simulink model "compilation_1_sm_computation"  (Simulink 7.8)
settings: Solver=ode4  StartTime=0.0  StopTime=inf  FixedStep=0.001  RelTol=1e-3
libraries: opal_lib x6
Description:
  | Model of a simple control system for use iin training.
settings Model: Creator=Paul Baracos  LastModifiedBy=emma
settings DataIOCC: SaveOutput=off  SaveTime=off  SignalLoggingName=sigsOut
settings OptimizationCC: BlockReduction=off  BooleanDataType=off  InlineInvariantSignals=on  InitFltsAndDblsToZero=on
settings DebuggingCC: SaveWithParameterizedLinksMsg=none  SignalResolutionControl=TryResolveAllWithWarning  SolverPrmCheckMsg=none  MultiTaskDSMMsg=warning  MultiTaskCondExecSysMsg=none  FcnCallInpInsideContextMsg=Use local settings  StrictBusMsg=None
settings HardwareCC: TargetUnknown=on
settings RTWCC: GenCodeOnly=on  IncludeERTFirstTime=on
settings GRTTargetCC: TargetFcnLib=ansi_tfl_tmw.mat

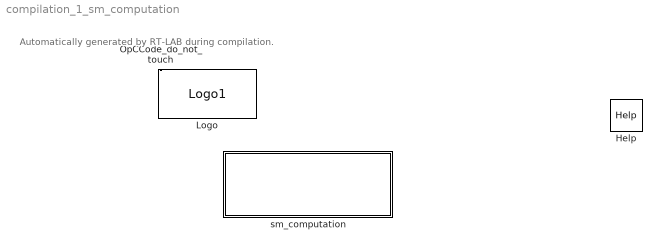
== system compilation_1_sm_computation ==
  note: Automatically generated by RT-LAB during compilation.
  Help : opal_lib/Help  docfile=../../help/help_compilation.html
  Logo : opal_lib/Logo1  vide=[]
  OpCCode_do_not_touch : opal_lib/Communication/OpCCode  SystemSampleTime=-1
  sm_computation : Subsystem

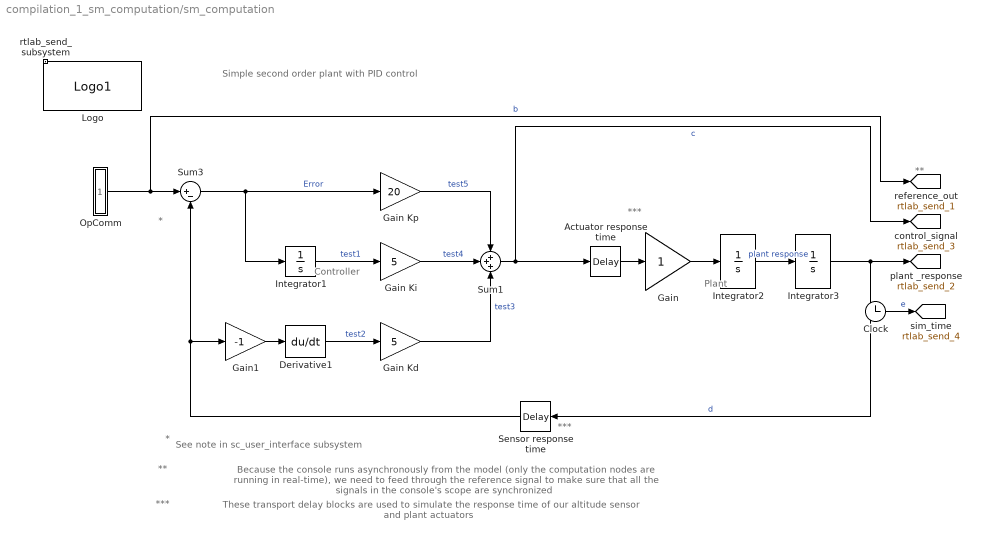
== system compilation_1_sm_computation/sm_computation ==
  note: Controller
  note: Plant
  note: Simple second order plant with PID control
  note: Because the console runs asynchronously from the model (only the computation nodes are running in real-time), we
      | need to feed through the reference signal to make sure that all the signals in the console's scope are synchronized
  note: **
  note: **
  note: *
  note: See note in sc_user_interface subsystem
  note: *
  note: ***
  note: These transport delay blocks are used to simulate the response time of our altitude sensor and plant actuators
  note: ***
  note: ***
  Actuator response time : TransportDelay  DelayTime=0.005
  Clock : Clock
  Derivative1 : Derivative
  Gain : Gain  SaturateOnIntegerOverflow=on  OutDataTypeStr=Inherit: Same as input  ParamDataTypeStr=Inherit: Same as input
  Gain Kd : Gain  Gain=5  SaturateOnIntegerOverflow=on  OutDataTypeStr=Inherit: Same as input  ParamDataTypeStr=Inherit: Same as input
  Gain Ki : Gain  Gain=5  SaturateOnIntegerOverflow=on  OutDataTypeStr=Inherit: Same as input  ParamDataTypeStr=Inherit: Same as input
  Gain Kp : Gain  Gain=20  SaturateOnIntegerOverflow=on  OutDataTypeStr=Inherit: Same as input  ParamDataTypeStr=Inherit: Same as input
  Gain1 : Gain  Gain=-1  SaturateOnIntegerOverflow=on  OutDataTypeStr=Inherit: Same as input  ParamDataTypeStr=Inherit: Same as input
  Integrator1 : Integrator
  Integrator2 : Integrator
  Integrator3 : Integrator  LimitOutput=on  UpperSaturationLimit=200  LowerSaturationLimit=0
  Logo : opal_lib/Logo1  vide=[]
  OpComm : Subsystem
      mask init:
      | opmaskdisplay('maskdisplay_block',gcb,'disp(''OpComm'')');
      mask Display:
      | patch([0 0.5 0.7 0],[1 1 0 0],[0.7 0.75 0.9]);
      | patch([1 0.53 0.73 1],[1 1 0 0],[1 0.8 0.7]);
      | plot([0 0 1 1 0],[0 1 1 0 0]);
      | disp('OpComm')
  Sensor response time : TransportDelay  DelayTime=0.005
  Sum1 : Sum  Inputs=+++  SaturateOnIntegerOverflow=on  InputSameDT=on  OutDataTypeStr=Inherit: Same as first input
  Sum3 : Sum  Inputs=|+-  SaturateOnIntegerOverflow=on  InputSameDT=on  OutDataTypeStr=Inherit: Same as first input
  rtlab_send_subsystem : Subsystem  Priority=-100
      mask Display: text(0,0,'');
  tag scope: rtlab_send_1=global, rtlab_send_2=global, rtlab_send_3=global, rtlab_send_4=global
  wires:
  OpComm/1(Out1) -> Sum3/1, [rtlab_send_1]  "b"
  Sum3/1 -> Gain Kp/1, Integrator1/1  "Error"
  Gain Kp/1 -> Sum1/1  "test5"
  Integrator1/1 -> Gain Ki/1  "test1"
  Derivative1/1 -> Gain Kd/1  "test2"
  Gain Ki/1 -> Sum1/2  "test4"
  Gain1/1 -> Derivative1/1
  Gain Kd/1 -> Sum1/3  "test3"
  Sum1/1 -> [rtlab_send_3], Actuator response time/1  "c"
  Sensor response time/1 -> Sum3/2, Gain1/1
  Integrator2/1 -> Integrator3/1  "plant response"
  Integrator3/1 -> [rtlab_send_2], Sensor response time/1  "d"
  Gain/1 -> Integrator2/1
  Actuator response time/1 -> Gain/1
  Clock/1 -> [rtlab_send_4]  "e"

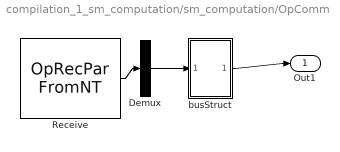
== system compilation_1_sm_computation/sm_computation/OpComm ==
  Demux : Demux  Outputs=[1]
  Receive : opal_lib/Communication/OpRecPar FromNT  Data_width=1  InitialConditions=93.5
  busStruct : Subsystem
  Out1 : Outport
  wires:
  Demux/1 -> busStruct/1(In1)
  busStruct/1(Out1) -> Out1/1
  Receive/1 -> Demux/1

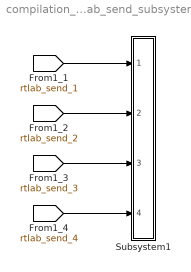
== system compilation_1_sm_computation/sm_computation/rtlab_send_subsystem ==
  Subsystem1 : Subsystem
  wires:
  [rtlab_send_1] -> Subsystem1/1(In1)
  [rtlab_send_2] -> Subsystem1/2(In2)
  [rtlab_send_3] -> Subsystem1/3(In3)
  [rtlab_send_4] -> Subsystem1/4(In4)

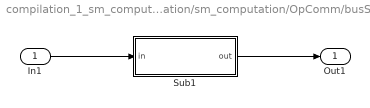
== system compilation_1_sm_computation/sm_computation/OpComm/busStruct ==
  In1 : Inport
  Sub1 : Subsystem
  Out1 : Outport
  wires:
  Sub1/1(out) -> Out1/1
  In1/1 -> Sub1/1(in)

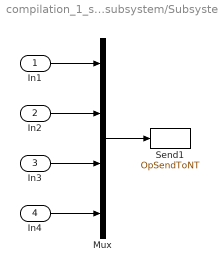
== system compilation_1_sm_computation/sm_computation/rtlab_send_subsystem/Subsystem1 ==
  In1 : Inport
  In2 : Inport  Port=2
  In3 : Inport  Port=3
  In4 : Inport  Port=4
  Mux : Mux
  Send1 : opal_lib/Communication/OpSendToNT  Acqu_group=1
  wires:
  Mux/1 -> Send1/1
  In1/1 -> Mux/1
  In2/1 -> Mux/2
  In3/1 -> Mux/3
  In4/1 -> Mux/4

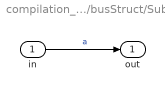
== system compilation_1_sm_computation/sm_computation/OpComm/busStruct/Sub1 ==
  in : Inport
  out : Outport
  wires:
  in/1 -> out/1  "a"
